simulink model "video_template"  (R2018a)
settings: Solver=VariableStepAuto  StartTime=0.0  StopTime=2/60  RelTol=1e-3
InitFcn:
  | I = imread('peppers.png');
  | height = 240;
  | width = 320;
  | Iresize = imresize(I, [height width]);
  | 
  | fps = 60;
  | f = fps * 402 * 324;
  | T = 1/f;
undefined symbols (not defined in the file): deltaTheta, maxRho, maxTheta
libraries: xbsIndex_r4 x18, hdlsllib x9, visionhdlio x2, simulink x1, dspswit3 x1, visionhdlutilities x1, dspvision x1, visionsources x1
settings Model: SimulationMode=accelerator  Creator=David Northcote  LastModifiedBy=David Northcote

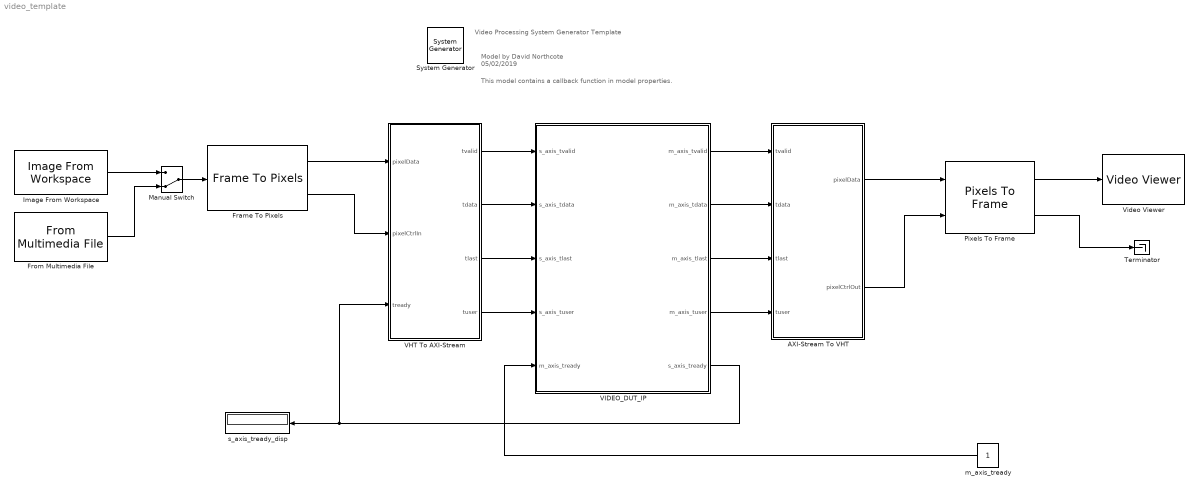
== system video_template ==
  note: This model contains a callback function in model properties.
  note: Model by David Northcote
      | 05/02/2019
  note: Video Processing System Generator Template
  " System Generator" : xbsIndex_r4/ System Generator  Tag=genX  xilinxfamily=zynq  part=xc7z020  speed=-1  package=clg400  synthesis_tool=Vivado  clock_wrapper=Clock Enables  directory=./netlist  proj_type=Vivado  Synth_file=Vivado Synthesis Defaults  Impl_file=Vivado Implementation Defaults  testbench=off  simulink_period=T  sysclk_period=T*1e9  dcm_input_clock_period=10  incr_netlist=off  trim_vbits=Everywhere in SubSystem  dbl_ovrd=According to Block Masks  core_generation=According to Block Masks  run_coregen=off  deprecated_control=off  eval_field=0  block_type=sysgen
  AXI-Stream To VHT : Subsystem  mask{height=height}
      mask prompts: height "Enter image height."
  Frame To Pixels : visionhdlio/Frame To Pixels  NumComponents=3  VideoFormat=240p  ActivePixelsPerLine=width  ActiveVideoLines=height  TotalPixelsPerLine=width  TotalVideoLines=height  StartingActiveLine=1  FrontPorch=0  SampleTime=0
      settings: SourceProductName=Vision HDL Toolbox  SourceProductBaseCode=VT
  From Multimedia File : dspvision/From Multimedia File  inputFilename=vipbarcode.mp4  loop=on  numPlays=inf  outputStreams=Video only  videoDataType=uint8  audioDataType=int16  inheritSampleTime=off  userDefinedSampleTime=1/60  noAudioOutput=off  isIntensityVideo=off  fourcc=RGB  colorVideoFormat=One multidimensional signal  outputEOF=off  dataOrg=Column-major  audioFrameSize=1024  computeAudioFrameSize=off  outSamplingMode=Sample based
      settings: SourceProductBaseCode=VP
  Image From Workspace : visionsources/Image From Workspace  Tag=vipblks_nd  ImageValue=Iresize  Ts=1/60  imagePorts=One multidimensional signal  OutPortLabels=R|G|B  ImageDataType=Inherit from 'Value'  Signed=on  WordLength=16  sdImageDataType=sfix(16)  FractionLengthMode=User-defined  FractionLength=15
      settings: SourceProductName=Computer Vision System Toolbox  SourceProductBaseCode=VP
  Manual Switch : ManualSwitch  CurrentSetting=0
  Pixels To Frame : visionhdlio/Pixels To Frame  NumComponents=3  VideoFormat=240p  ActivePixelsPerLine=maxRho*2  ActiveVideoLines=maxTheta+deltaTheta  TotalPixelsPerLine=maxRho*2  TotalVideoLines=maxTheta+deltaTheta
      settings: SourceProductName=Vision HDL Toolbox  SourceProductBaseCode=VT
  Terminator : Terminator
  VHT To AXI-Stream : Subsystem
  VIDEO_DUT_IP : Subsystem
  Video Viewer : VideoViewer  FigPos=[2034 678 418 304]
  m_axis_tready : Constant  VectorParams1D=off  SampleTime=-1
  s_axis_tready_disp : Display
  wires:
  VIDEO_DUT_IP/5(s_axis_tready) -> s_axis_tready_disp/1, VHT To AXI-Stream/3(tready)
  VHT To AXI-Stream/1(tvalid) -> VIDEO_DUT_IP/1(s_axis_tvalid)
  VHT To AXI-Stream/2(tdata) -> VIDEO_DUT_IP/2(s_axis_tdata)
  VHT To AXI-Stream/3(tlast) -> VIDEO_DUT_IP/3(s_axis_tlast)
  VHT To AXI-Stream/4(tuser) -> VIDEO_DUT_IP/4(s_axis_tuser)
  m_axis_tready/1 -> VIDEO_DUT_IP/5(m_axis_tready)
  Frame To Pixels/1 -> VHT To AXI-Stream/1(pixelData)
  Frame To Pixels/2 -> VHT To AXI-Stream/2(pixelCtrlIn)
  VIDEO_DUT_IP/4(m_axis_tuser) -> AXI-Stream To VHT/4(tuser)
  VIDEO_DUT_IP/3(m_axis_tlast) -> AXI-Stream To VHT/3(tlast)
  VIDEO_DUT_IP/2(m_axis_tdata) -> AXI-Stream To VHT/2(tdata)
  VIDEO_DUT_IP/1(m_axis_tvalid) -> AXI-Stream To VHT/1(tvalid)
  AXI-Stream To VHT/1(pixelData) -> Pixels To Frame/1
  AXI-Stream To VHT/2(pixelCtrlOut) -> Pixels To Frame/2
  Pixels To Frame/1 -> Video Viewer/1
  Pixels To Frame/2 -> Terminator/1
  Manual Switch/1 -> Frame To Pixels/1
  Image From Workspace/1 -> Manual Switch/1
  From Multimedia File/1 -> Manual Switch/2

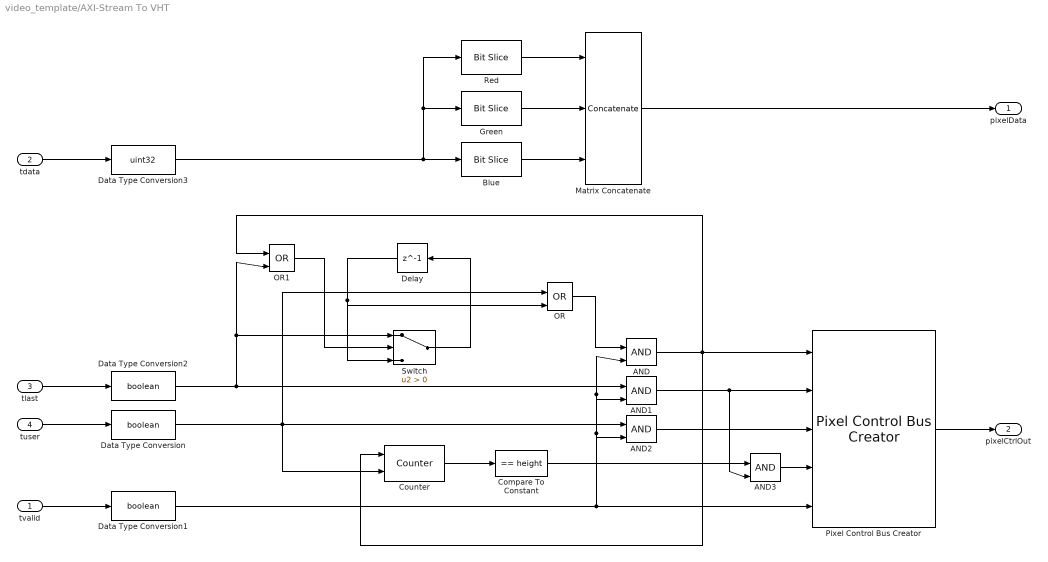
== system video_template/AXI-Stream To VHT ==
  tvalid : Inport
  tdata : Inport  Port=2
  tlast : Inport  Port=3
  tuser : Inport  Port=4
  AND{,1..3} (4 alike) : Logic  IconShape=distinctive  AllPortsSameDT=off  OutDataTypeStr=boolean
  Blue : hdlsllib/Logic and Bit Operations/Bit Slice  lidx=15  ridx=8
  Compare To Constant : simulink/Logic and Bit Operations/Compare To Constant  relop===  const=height  OutDataTypeStr=boolean
  Counter : dspswit3/Counter  Direction=Up  CountEvent=Non-zero sample  CounterSize=32 bits  MaxCount=255  InitialCount=0  Output=Count  HitValue=32  ResetInput=on  SamplesPerFrame=1  Ts=1  CntDtype=uint32  HitDtype=Logical
  Data Type Conversion : DataTypeConversion  OutDataTypeStr=boolean
  Data Type Conversion1 : DataTypeConversion  OutDataTypeStr=boolean
  Data Type Conversion2 : DataTypeConversion  OutDataTypeStr=boolean
  Data Type Conversion3 : DataTypeConversion  OutDataTypeStr=uint32
  Delay : Delay  DelayLength=1
  Green : hdlsllib/Logic and Bit Operations/Bit Slice  lidx=7  ridx=0
  Matrix Concatenate : Concatenate  NumInputs=3  Mode=Multidimensional array  ConcatenateDimension=2
  OR : Logic  Operator=OR  IconShape=distinctive  AllPortsSameDT=off  OutDataTypeStr=boolean
  OR1 : Logic  Operator=OR  IconShape=distinctive  AllPortsSameDT=off  OutDataTypeStr=boolean
  Pixel Control Bus Creator : visionhdlutilities/Pixel Control Bus Creator
      settings: SourceProductName=Vision HDL Toolbox  SourceProductBaseCode=VT
  Red : hdlsllib/Logic and Bit Operations/Bit Slice  lidx=23  ridx=16
  Switch : Switch  Criteria=u2 > Threshold
  pixelData : Outport
  pixelCtrlOut : Outport  Port=2
  wires:
  tdata/1 -> Data Type Conversion3/1
  Pixel Control Bus Creator/1 -> pixelCtrlOut/1
  tuser/1 -> Data Type Conversion/1
  tlast/1 -> Data Type Conversion2/1
  tvalid/1 -> Data Type Conversion1/1
  Counter/1 -> Compare To Constant/1
  Data Type Conversion2/1 -> AND1/1, OR1/2, Switch/1
  Data Type Conversion1/1 -> AND2/2, AND1/2, AND/2, Pixel Control Bus Creator/5
  Data Type Conversion/1 -> Counter/2, AND2/1, OR/1
  OR/1 -> AND/1
  Switch/1 -> Delay/1
  Delay/1 -> OR/2, Switch/3
  OR1/1 -> Switch/2
  AND/1 -> Counter/1, OR1/1, Pixel Control Bus Creator/1
  AND2/1 -> Pixel Control Bus Creator/3
  Compare To Constant/1 -> AND3/1
  AND1/1 -> AND3/2, Pixel Control Bus Creator/2
  AND3/1 -> Pixel Control Bus Creator/4
  Matrix Concatenate/1 -> pixelData/1
  Green/1 -> Matrix Concatenate/2
  Blue/1 -> Matrix Concatenate/3
  Red/1 -> Matrix Concatenate/1
  Data Type Conversion3/1 -> Red/1, Green/1, Blue/1

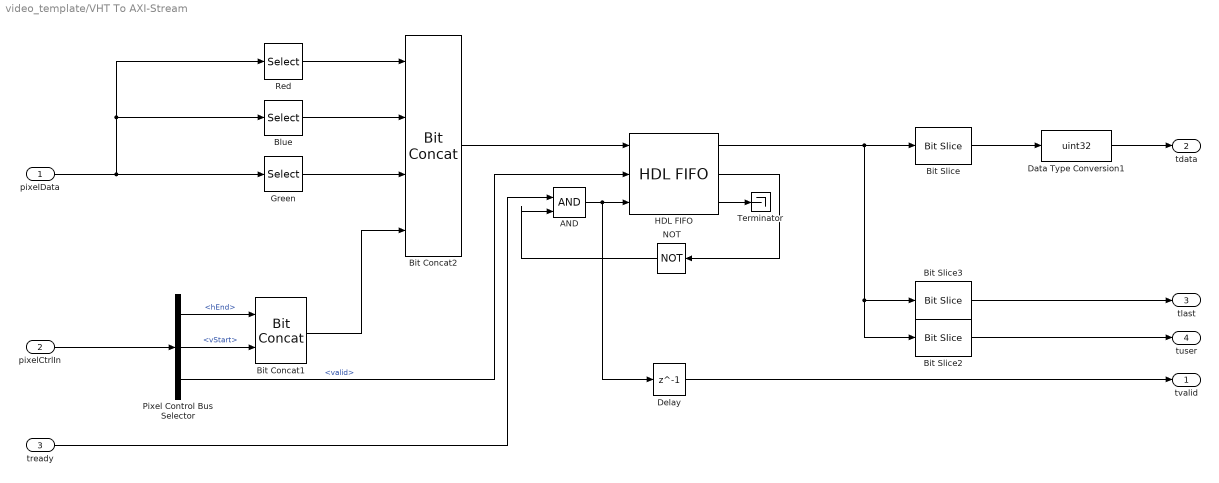
== system video_template/VHT To AXI-Stream ==
  pixelData : Inport
  pixelCtrlIn : Inport  Port=2
  tready : Inport  Port=3
  AND : Logic  IconShape=distinctive  AllPortsSameDT=off  OutDataTypeStr=boolean
  Bit Concat1 : hdlsllib/Logic and Bit Operations/Bit Concat  numInputs=2
      settings: SourceProductName=HDL Coder  SourceProductBaseCode=HD
  Bit Concat2 : hdlsllib/Logic and Bit Operations/Bit Concat  numInputs=4
      settings: SourceProductName=HDL Coder  SourceProductBaseCode=HD
  Bit Slice : hdlsllib/Logic and Bit Operations/Bit Slice  lidx=25  ridx=2
  Bit Slice2 : hdlsllib/Logic and Bit Operations/Bit Slice  lidx=0  ridx=0
  Bit Slice3 : hdlsllib/Logic and Bit Operations/Bit Slice  lidx=1  ridx=1
  Blue : Selector  InputPortWidth=3  IndexOptions=Index vector (dialog)  Indices=3  OutputSizes=1
  Data Type Conversion1 : DataTypeConversion  OutDataTypeStr=uint32
  Delay : Delay  DelayLength=1
  Green : Selector  InputPortWidth=3  IndexOptions=Index vector (dialog)  Indices=2  OutputSizes=1
  HDL FIFO : hdlsllib/HDL RAMs/HDL FIFO  fifo_size=1024  ratio=1  push_msg=Error  pop_msg=Error  show_empty=on  show_full=on  show_num=off
      settings: SourceProductName=HDL Coder  SourceProductBaseCode=HD
  NOT : Logic  Operator=NOT  IconShape=distinctive  AllPortsSameDT=off  OutDataTypeStr=boolean
  Pixel Control Bus Selector : BusSelector  OutputSignals=hEnd,vStart,valid
  Red : Selector  InputPortWidth=3  IndexOptions=Index vector (dialog)  Indices=1  OutputSizes=1
  Terminator : Terminator
  tvalid : Outport
  tdata : Outport  Port=2
  tlast : Outport  Port=3
  tuser : Outport  Port=4
  wires:
  pixelCtrlIn/1 -> Pixel Control Bus Selector/1
  Bit Concat2/1 -> HDL FIFO/1
  tready/1 -> AND/1
  HDL FIFO/2 -> NOT/1
  NOT/1 -> AND/2
  Bit Slice3/1 -> tlast/1
  Bit Slice2/1 -> tuser/1
  AND/1 -> Delay/1, HDL FIFO/3
  Pixel Control Bus Selector/1 -> Bit Concat1/1  "<hEnd>"
  Pixel Control Bus Selector/2 -> Bit Concat1/2  "<vStart>"
  Pixel Control Bus Selector/3 -> HDL FIFO/2  "<valid>"
  Delay/1 -> tvalid/1
  HDL FIFO/3 -> Terminator/1
  Bit Concat1/1 -> Bit Concat2/4
  pixelData/1 -> Red/1, Blue/1, Green/1
  Bit Slice/1 -> Data Type Conversion1/1
  HDL FIFO/1 -> Bit Slice/1, Bit Slice3/1, Bit Slice2/1
  Data Type Conversion1/1 -> tdata/1
  Blue/1 -> Bit Concat2/2
  Green/1 -> Bit Concat2/3
  Red/1 -> Bit Concat2/1

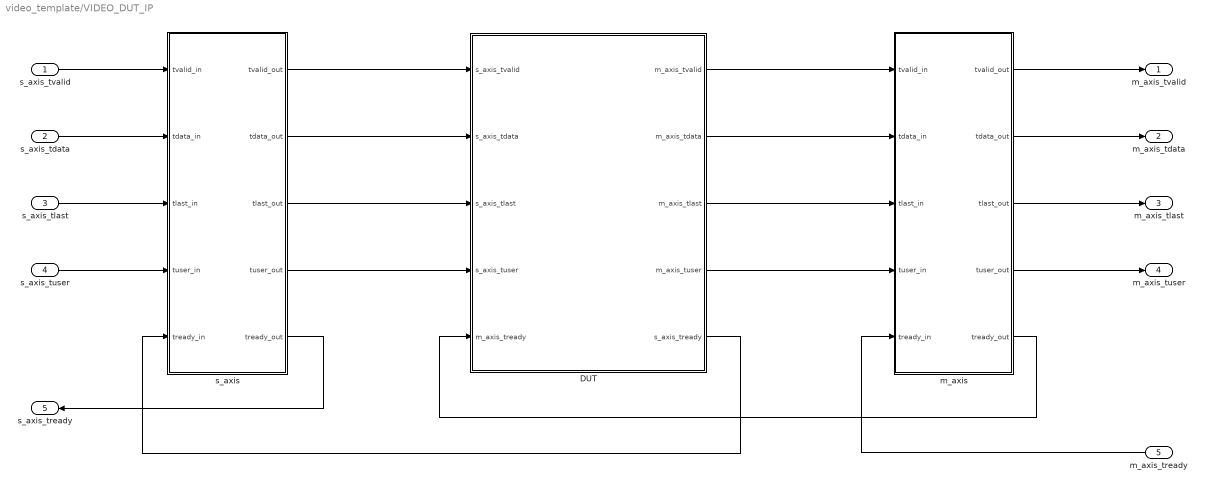
== system video_template/VIDEO_DUT_IP ==
  s_axis_tvalid : Inport
  s_axis_tdata : Inport  Port=2
  s_axis_tlast : Inport  Port=3
  s_axis_tuser : Inport  Port=4
  m_axis_tready : Inport  Port=5
  DUT : Subsystem
  m_axis : Subsystem
  s_axis : Subsystem
  m_axis_tvalid : Outport
  m_axis_tdata : Outport  Port=2
  m_axis_tlast : Outport  Port=3
  m_axis_tuser : Outport  Port=4
  s_axis_tready : Outport  Port=5
  wires:
  s_axis/4(tuser_out) -> DUT/4(s_axis_tuser)
  m_axis/2(tdata_out) -> m_axis_tdata/1
  s_axis/1(tvalid_out) -> DUT/1(s_axis_tvalid)
  DUT/2(m_axis_tdata) -> m_axis/2(tdata_in)
  s_axis/3(tlast_out) -> DUT/3(s_axis_tlast)
  DUT/1(m_axis_tvalid) -> m_axis/1(tvalid_in)
  DUT/5(s_axis_tready) -> s_axis/5(tready_in)
  s_axis/2(tdata_out) -> DUT/2(s_axis_tdata)
  DUT/3(m_axis_tlast) -> m_axis/3(tlast_in)
  DUT/4(m_axis_tuser) -> m_axis/4(tuser_in)
  m_axis/5(tready_out) -> DUT/5(m_axis_tready)
  m_axis/4(tuser_out) -> m_axis_tuser/1
  m_axis/3(tlast_out) -> m_axis_tlast/1
  s_axis/5(tready_out) -> s_axis_tready/1
  m_axis/1(tvalid_out) -> m_axis_tvalid/1
  s_axis_tvalid/1 -> s_axis/1(tvalid_in)
  s_axis_tdata/1 -> s_axis/2(tdata_in)
  m_axis_tready/1 -> m_axis/5(tready_in)
  s_axis_tlast/1 -> s_axis/3(tlast_in)
  s_axis_tuser/1 -> s_axis/4(tuser_in)

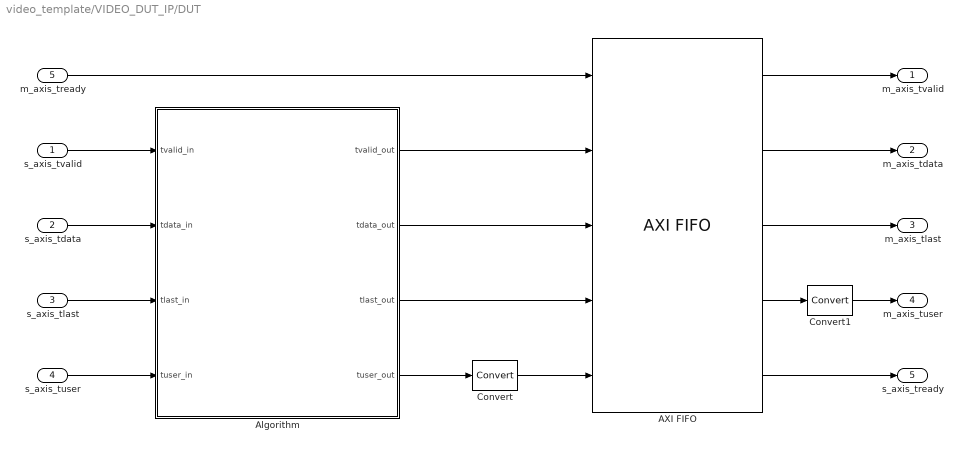
== system video_template/VIDEO_DUT_IP/DUT ==
  s_axis_tvalid : Inport
  s_axis_tdata : Inport  Port=2
  s_axis_tlast : Inport  Port=3
  s_axis_tuser : Inport  Port=4
  m_axis_tready : Inport  Port=5
  AXI FIFO : xbsIndex_r4/AXI FIFO  input_depth_axis=128  actual_fifo_depth_label=130  enable_tdata=on  enable_tdest=off  enable_tstrb=off  enable_tready=on  enable_tid=off  enable_tuser=on  enable_tkeep=off  enable_tlast=on  has_aresetn=off  enable_data_counts_axis=off  fifo_implementation_type_axis=Common Clock Distributed RAM  trim_axipin_name=on  programmable_full_type_axis=Full  full_threshold_assert_value_axis=0  programmable_empty_type_axis=Empty  empty_threshold_assert_value_axis=1022  underflow_flag_axi=0  underflow_sense_axi=Active High  overflow_flag_axi=0  overflow_sense_axi=Active High  block_type=axi_fifo
  Algorithm : Subsystem
  Convert : xbsIndex_r4/Convert  gui_display_data_type=Fixed-point  arith_type=Unsigned  n_bits=1  bin_pt=0  float_type=Single  exp_bits=8  fraction_bits=24  quantization=Truncate  overflow=Wrap  en=off  latency=0  pipeline=off  dbl_ovrd=off  block_type=convert
  Convert1 : xbsIndex_r4/Convert  gui_display_data_type=Boolean  arith_type=Boolean  n_bits=1  bin_pt=0  float_type=Single  exp_bits=8  fraction_bits=24  quantization=Truncate  overflow=Wrap  en=off  latency=0  pipeline=off  dbl_ovrd=off  block_type=convert
  m_axis_tvalid : Outport
  m_axis_tdata : Outport  Port=2
  m_axis_tlast : Outport  Port=3
  m_axis_tuser : Outport  Port=4
  s_axis_tready : Outport  Port=5
  wires:
  AXI FIFO/5 -> s_axis_tready/1
  AXI FIFO/2 -> m_axis_tdata/1
  AXI FIFO/3 -> m_axis_tlast/1
  Algorithm/3(tlast_out) -> AXI FIFO/4
  Algorithm/1(tvalid_out) -> AXI FIFO/2
  AXI FIFO/4 -> Convert1/1
  AXI FIFO/1 -> m_axis_tvalid/1
  Algorithm/2(tdata_out) -> AXI FIFO/3
  Algorithm/4(tuser_out) -> Convert/1
  s_axis_tdata/1 -> Algorithm/2(tdata_in)
  s_axis_tuser/1 -> Algorithm/4(tuser_in)
  s_axis_tvalid/1 -> Algorithm/1(tvalid_in)
  s_axis_tlast/1 -> Algorithm/3(tlast_in)
  m_axis_tready/1 -> AXI FIFO/1
  Convert/1 -> AXI FIFO/5
  Convert1/1 -> m_axis_tuser/1

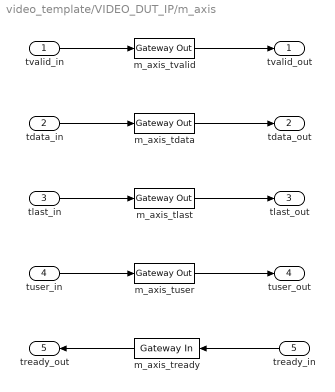
== system video_template/VIDEO_DUT_IP/m_axis ==
  tvalid_in : Inport
  tdata_in : Inport  Port=2
  tlast_in : Inport  Port=3
  tuser_in : Inport  Port=4
  tready_in : Inport  Port=5
  m_axis_tdata : xbsIndex_r4/Gateway Out  inherit_from_input=on  hdl_port=on  rows=1  columns=1  UseAsDAC=off  DACChannel='1'  interface=None  automatic_assignment=on  address_offset=hex2dec('00')  intf_name=''  intf_description=''  timing_constraint=None  locs_specified=off  LOCs={}  io_standard={}  block_type=gatewayout
  m_axis_tlast : xbsIndex_r4/Gateway Out  inherit_from_input=on  hdl_port=on  rows=1  columns=1  UseAsDAC=off  DACChannel='1'  interface=None  automatic_assignment=on  address_offset=hex2dec('00')  intf_name=''  intf_description=''  timing_constraint=None  locs_specified=off  LOCs={}  io_standard={}  block_type=gatewayout
  m_axis_tready : xbsIndex_r4/Gateway In  gui_display_data_type=Boolean  arith_type=Boolean  n_bits=16  bin_pt=14  preci_type=Single  exp_width=8  frac_width=24  rows=1  columns=1  quantization="Round  (unbiased: +/- Inf)"  overflow=Saturate  period=T  UseAsADC=off  ADCChannel='1'  interface=None  automatic_assignment=on  address_offset=hex2dec('00')  intf_name=''  intf_description=''  default_value=0  timing_constraint=None  locs_specified=off  LOCs={}  io_standard={}  inherit_from_input=off  hdl_port=on  dbl_ovrd=off  block_type=gatewayin
  m_axis_tuser : xbsIndex_r4/Gateway Out  inherit_from_input=on  hdl_port=on  rows=1  columns=1  UseAsDAC=off  DACChannel='1'  interface=None  automatic_assignment=on  address_offset=hex2dec('00')  intf_name=''  intf_description=''  timing_constraint=None  locs_specified=off  LOCs={}  io_standard={}  block_type=gatewayout
  m_axis_tvalid : xbsIndex_r4/Gateway Out  inherit_from_input=on  hdl_port=on  rows=1  columns=1  UseAsDAC=off  DACChannel='1'  interface=None  automatic_assignment=on  address_offset=hex2dec('00')  intf_name=''  intf_description=''  timing_constraint=None  locs_specified=off  LOCs={}  io_standard={}  block_type=gatewayout
  tvalid_out : Outport
  tdata_out : Outport  Port=2
  tlast_out : Outport  Port=3
  tuser_out : Outport  Port=4
  tready_out : Outport  Port=5
  wires:
  m_axis_tuser/1 -> tuser_out/1
  tlast_in/1 -> m_axis_tlast/1
  tuser_in/1 -> m_axis_tuser/1
  tvalid_in/1 -> m_axis_tvalid/1
  m_axis_tready/1 -> tready_out/1
  m_axis_tdata/1 -> tdata_out/1
  m_axis_tlast/1 -> tlast_out/1
  tdata_in/1 -> m_axis_tdata/1
  tready_in/1 -> m_axis_tready/1
  m_axis_tvalid/1 -> tvalid_out/1

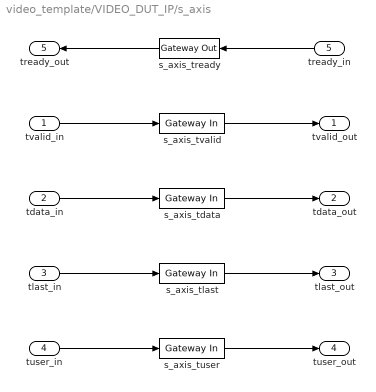
== system video_template/VIDEO_DUT_IP/s_axis ==
  tvalid_in : Inport
  tdata_in : Inport  Port=2
  tlast_in : Inport  Port=3
  tuser_in : Inport  Port=4
  tready_in : Inport  Port=5
  s_axis_tdata : xbsIndex_r4/Gateway In  gui_display_data_type=Fixed-point  arith_type=Unsigned  n_bits=32  bin_pt=0  preci_type=Single  exp_width=8  frac_width=24  rows=1  columns=1  quantization="Round  (unbiased: +/- Inf)"  overflow=Saturate  period=T  UseAsADC=off  ADCChannel='1'  interface=None  automatic_assignment=on  address_offset=hex2dec('00')  intf_name=''  intf_description=''  default_value=0  timing_constraint=None  locs_specified=off  LOCs={}  io_standard={}  inherit_from_input=off  hdl_port=on  dbl_ovrd=off  block_type=gatewayin
  s_axis_tlast : xbsIndex_r4/Gateway In  gui_display_data_type=Boolean  arith_type=Boolean  n_bits=16  bin_pt=14  preci_type=Single  exp_width=8  frac_width=24  rows=1  columns=1  quantization="Round  (unbiased: +/- Inf)"  overflow=Saturate  period=T  UseAsADC=off  ADCChannel='1'  interface=None  automatic_assignment=on  address_offset=hex2dec('00')  intf_name=''  intf_description=''  default_value=0  timing_constraint=None  locs_specified=off  LOCs={}  io_standard={}  inherit_from_input=off  hdl_port=on  dbl_ovrd=off  block_type=gatewayin
  s_axis_tready : xbsIndex_r4/Gateway Out  inherit_from_input=on  hdl_port=on  rows=1  columns=1  UseAsDAC=off  DACChannel='1'  interface=None  automatic_assignment=on  address_offset=hex2dec('00')  intf_name=''  intf_description=''  timing_constraint=None  locs_specified=off  LOCs={}  io_standard={}  block_type=gatewayout
  s_axis_tuser : xbsIndex_r4/Gateway In  gui_display_data_type=Boolean  arith_type=Boolean  n_bits=16  bin_pt=14  preci_type=Single  exp_width=8  frac_width=24  rows=1  columns=1  quantization="Round  (unbiased: +/- Inf)"  overflow=Saturate  period=T  UseAsADC=off  ADCChannel='1'  interface=None  automatic_assignment=on  address_offset=hex2dec('00')  intf_name=''  intf_description=''  default_value=0  timing_constraint=None  locs_specified=off  LOCs={}  io_standard={}  inherit_from_input=off  hdl_port=on  dbl_ovrd=off  block_type=gatewayin
  s_axis_tvalid : xbsIndex_r4/Gateway In  gui_display_data_type=Boolean  arith_type=Boolean  n_bits=16  bin_pt=14  preci_type=Single  exp_width=8  frac_width=24  rows=1  columns=1  quantization="Round  (unbiased: +/- Inf)"  overflow=Saturate  period=T  UseAsADC=off  ADCChannel='1'  interface=None  automatic_assignment=on  address_offset=hex2dec('00')  intf_name=''  intf_description=''  default_value=0  timing_constraint=None  locs_specified=off  LOCs={}  io_standard={}  inherit_from_input=off  hdl_port=on  dbl_ovrd=off  block_type=gatewayin
  tvalid_out : Outport
  tdata_out : Outport  Port=2
  tlast_out : Outport  Port=3
  tuser_out : Outport  Port=4
  tready_out : Outport  Port=5
  wires:
  tready_in/1 -> s_axis_tready/1
  s_axis_tdata/1 -> tdata_out/1
  tdata_in/1 -> s_axis_tdata/1
  s_axis_tready/1 -> tready_out/1
  tlast_in/1 -> s_axis_tlast/1
  tuser_in/1 -> s_axis_tuser/1
  s_axis_tlast/1 -> tlast_out/1
  s_axis_tuser/1 -> tuser_out/1
  tvalid_in/1 -> s_axis_tvalid/1
  s_axis_tvalid/1 -> tvalid_out/1

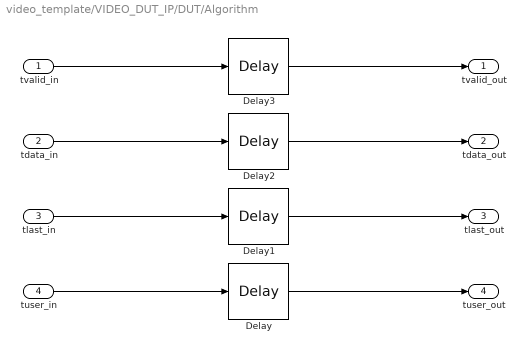
== system video_template/VIDEO_DUT_IP/DUT/Algorithm ==
  tvalid_in : Inport
  tdata_in : Inport  Port=2
  tlast_in : Inport  Port=3
  tuser_in : Inport  Port=4
  Delay{,1..3} (4 alike) : xbsIndex_r4/Delay  rst=off  infoeditControl=Selection of Reset will increase slice count due to use of real FFs and instead of SRLs  en=off  latency=1  reg_retiming=off  dbl_ovrd=off  block_type=delay
  tvalid_out : Outport
  tdata_out : Outport  Port=2
  tlast_out : Outport  Port=3
  tuser_out : Outport  Port=4
  wires:
  Delay/1 -> tuser_out/1
  Delay2/1 -> tdata_out/1
  tvalid_in/1 -> Delay3/1
  tuser_in/1 -> Delay/1
  Delay3/1 -> tvalid_out/1
  Delay1/1 -> tlast_out/1
  tdata_in/1 -> Delay2/1
  tlast_in/1 -> Delay1/1
